simulink model "Lab5Pt1Correct"  (R2020b)
settings: Solver=ode3  StartTime=0.0  StopTime=1510  RelTol=1e-3  EnableMultiTasking=on
undefined symbols (not defined in the file or in its folder): f
settings Model: Creator=Mukhtar Hussain  LastModifiedBy=abenkum
settings SolverCC: AutoInsertRateTranBlk=on
settings DataIOCC: LimitDataPoints=on  SaveFormat=Array  ReturnWorkspaceOutputs=off
settings OptimizationCC: LifeSpan=inf
settings DebuggingCC: SolverPrmCheckMsg=warning  SFUnexpectedBacktrackingDiag=warning  SFNoUnconditionalDefaultTransitionDiag=warning  SFExecutionAtInitializationDiag=none  ArithmeticOperatorsInVariantConditions=warning
settings HardwareCC: ProdBitPerPointer=32  ProdBitPerSizeT=32  ProdBitPerPtrDiffT=32  ProdLargestAtomicFloat=None  ProdIntDivRoundTo=Undefined  ProdEndianess=Unspecified  ProdWordSize=32  ProdHWDeviceType=32-bit Generic
settings ModelReferenceCC: PropagateSignalLabelsOutOfModel=off
settings SFSimCC: SimUseLocalCustomCode=off  CustomCodeUndefinedFunction=UseInterfaceOnly
settings RTWCC: RTWUseLocalCustomCode=off
settings CodeAppCC: StateflowObjectComments=on
settings GRTTargetCC: TargetLangStandard=C89/C90 (ANSI)
settings ConfigComp: CovMetricSettings=dw  CovSaveCumulativeToWorkspaceVar=on  CovSaveSingleToWorkspaceVar=on  CovExternalEMLEnable=off  CovSFcnEnable=off

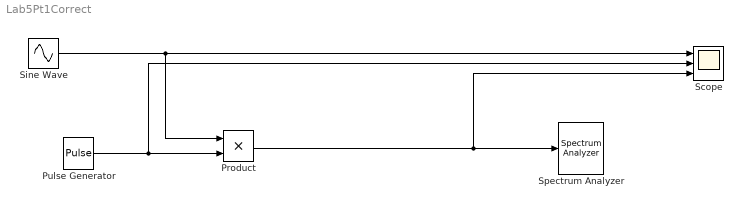
== system Lab5Pt1Correct ==
  Product : Product
  Pulse Generator : DiscretePulseGenerator  Period=100  SampleTime=0.001
  Scope : Scope  NumInputPorts=3
  Sine Wave : Sin  SineType=Sample based  Frequency=2*pi*f  Phase=pi/2  Samples=125  SampleTime=0.001
  Spectrum Analyzer : SpectrumAnalyzer
  wires:
  Pulse Generator/1 -> Scope/2, Product/2
  Sine Wave/1 -> Product/1, Scope/1
  Product/1 -> Spectrum Analyzer/1, Scope/3
